simulink model "szabalyozo2"  (R2021a)
settings: Solver=VariableStepAuto  StartTime=0.0  StopTime=0.5  RelTol=1e-3
values from neighbouring files (symbols this model uses):
  Ad = [-0.6 -2 ... (first row only)    [folyamat.m]    (also in szamol.m = tetam(1:2,1:2)')
  Bd = [1 0 ... (first row only)    [folyamat.m]    (also in szamol.m = tetam(3:4,:)')
  Cd = [1 -1]    [folyamat.m]    (also in szamol.m)
  teta = teta+K*e    [becslo.m]    (also in folyamat.m = [Ad' ; Bd'])
settings Model: Creator=Krisz  LastModifiedBy=Krisz

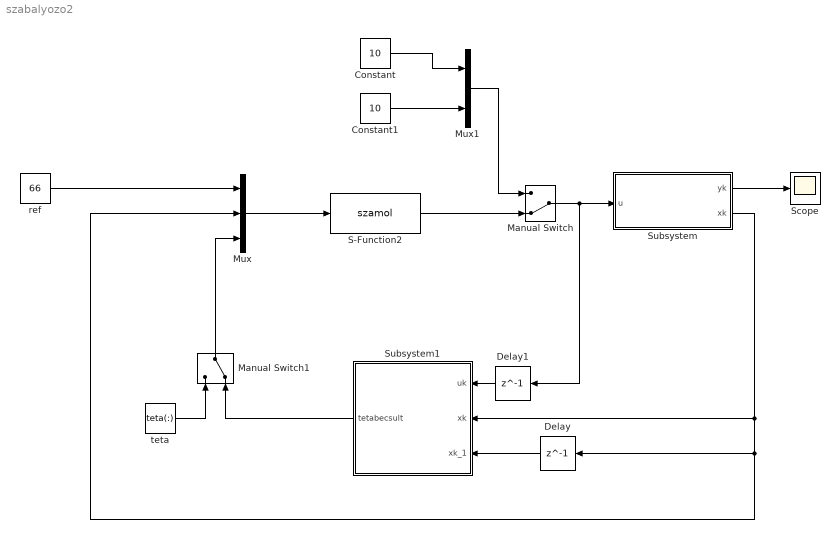
== system szabalyozo2 ==
  Constant : Constant  Value=10
  Constant1 : Constant  Value=10
  Delay : Delay  DelayLength=1  InitialCondition=0
  Delay1 : Delay  DelayLength=1  InitialCondition=0
  Manual Switch : ManualSwitch  CurrentSetting=0
  Manual Switch1 : ManualSwitch  CurrentSetting=0
  Mux : Mux  Inputs=3
  Mux1 : Mux  Inputs=2
  S-Function2 : S-Function  FunctionName=szamol  SFunctionDeploymentMode=off  EnableBusSupport=off
  Scope : Scope
  Subsystem : Subsystem  mask{Ad=Ad, Bd=Bd, Cd=Cd}
  Subsystem1 : Subsystem  mask{Ad=Ad, Bd=Bd, Cd=Cd}
  ref : Constant  Value=66
  teta : Constant  Value=teta(:)
  wires:
  Manual Switch/1 -> Delay1/1, Subsystem/1(u)
  Subsystem/1(yk) -> Scope/1
  Subsystem/2(xk) -> Subsystem1/2(xk), Mux/2, Delay/1
  ref/1 -> Mux/1
  Mux/1 -> S-Function2/1
  S-Function2/1 -> Manual Switch/2
  Constant/1 -> Mux1/1
  Constant1/1 -> Mux1/2
  Mux1/1 -> Manual Switch/1
  Delay/1 -> Subsystem1/3(xk_1)
  Subsystem1/1(tetabecsult) -> Manual Switch1/2
  teta/1 -> Manual Switch1/1
  Manual Switch1/1 -> Mux/3
  Delay1/1 -> Subsystem1/1(uk)

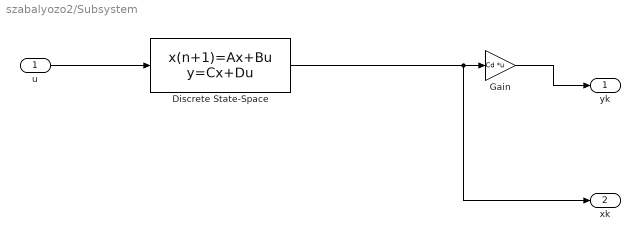
== system szabalyozo2/Subsystem ==
  u : Inport
  Discrete State-Space : DiscreteStateSpace  A=Ad  B=Bd  C=eye(2)  D=zeros(2,2)  SampleTime=-1
  Gain : Gain  Gain=Cd  Multiplication=Matrix(K*u)
  yk : Outport
  xk : Outport  Port=2
  wires:
  Discrete State-Space/1 -> Gain/1, xk/1
  u/1 -> Discrete State-Space/1
  Gain/1 -> yk/1

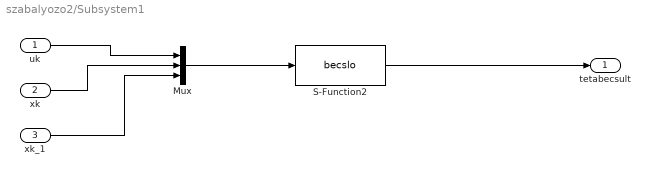
== system szabalyozo2/Subsystem1 ==
  uk : Inport
  xk : Inport  Port=2
  xk_1 : Inport  Port=3
  Mux : Mux  Inputs=3
  S-Function2 : S-Function  FunctionName=becslo  SFunctionDeploymentMode=off  EnableBusSupport=off
  tetabecsult : Outport
  wires:
  uk/1 -> Mux/1
  xk/1 -> Mux/2
  Mux/1 -> S-Function2/1
  S-Function2/1 -> tetabecsult/1
  xk_1/1 -> Mux/3
